simulink model "jellystone_v3"  (R2016b)
settings: Solver=FixedStepAuto  StartTime=0.0  StopTime=30  FixedStep=.2  RelTol=1e-3
settings Model: Creator=thomaskennedy  LastModifiedBy=thomaskennedy

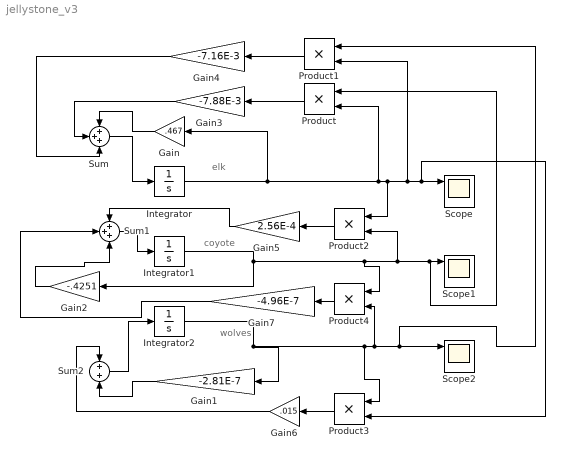
== system jellystone_v3 ==
  note: elk
  note: coyote
  note: wolves
  Gain : Gain  Gain=.467
  Gain1 : Gain  Gain=-2.81E-7
  Gain2 : Gain  Gain=-.4251
  Gain3 : Gain  Gain=-7.88E-3
  Gain4 : Gain  Gain=-7.16E-3
  Gain5 : Gain  Gain=2.56E-4
  Gain6 : Gain  Gain=.015
  Gain7 : Gain  Gain=-4.96E-7
  Integrator : Integrator  InitialCondition=311.217
  Integrator1 : Integrator  InitialCondition=800
  Integrator2 : Integrator  InitialCondition=1
  Product{,1..4} (5 alike) : Product
  Scope : Scope  NumInputPorts=3
  Scope1 : Scope  NumInputPorts=3
  Scope2 : Scope  NumInputPorts=3
  Sum : Sum  Inputs=3
  Sum1 : Sum  Inputs=3
  Sum2 : Sum  Inputs=2
  wires:
  Integrator1/1 -> Gain2/1, Product4/1, Product2/2, Product/1, Scope1/1
  Integrator2/1 -> Product3/1, Product4/2, Product1/1, Scope2/1, Gain1/1
  Product/1 -> Gain3/1
  Gain/1 -> Sum/1
  Sum/1 -> Integrator/1
  Gain3/1 -> Sum/2
  Product1/1 -> Gain4/1
  Gain4/1 -> Sum/3
  Gain2/1 -> Sum1/3
  Sum1/1 -> Integrator1/1
  Product2/1 -> Gain5/1
  Gain5/1 -> Sum1/1
  Gain1/1 -> Sum2/2
  Sum2/1 -> Integrator2/1
  Integrator/1 -> Gain/1, Product/2, Product2/1, Product1/2, Product3/2, Scope/1
  Product3/1 -> Gain6/1
  Gain6/1 -> Sum2/1
  Product4/1 -> Gain7/1
  Gain7/1 -> Sum1/2
